simulink model "ClosedLoop_Test"  (R2024a)
settings: Solver=VariableStepAuto  StartTime=0.0  StopTime=10.0  RelTol=1e-3
libraries: RCTblocks x7
settings Model: Creator=Thoma  LastModifiedBy=Thoma

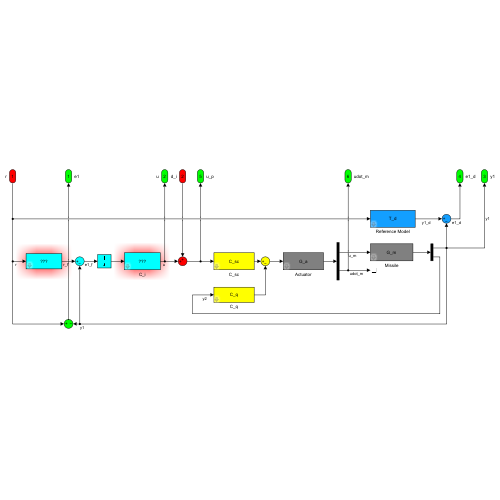
[thumbnail: Simulink's stored preview of the top-level diagram]
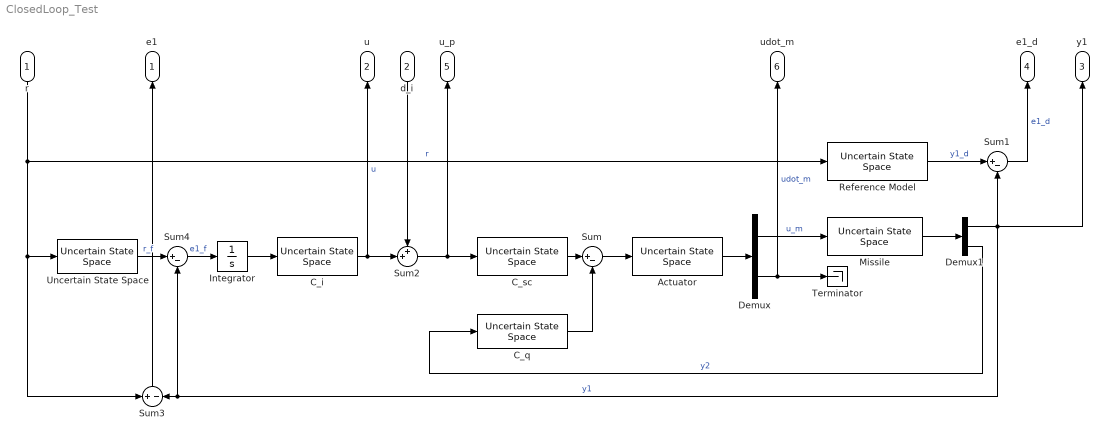
== system ClosedLoop_Test ==
  r : Inport
  d_i : Inport  Port=2
  Actuator : RCTblocks/Uncertain State Space  Tag=USS  USystem=G_a  UValue=[]  X0=[]  uX0=[]
  C_i : RCTblocks/Uncertain State Space  Tag=USS  USystem=C_i  UValue=[]  X0=[]  uX0=[]
  C_q : RCTblocks/Uncertain State Space  Tag=USS  USystem=C_q  UValue=[]  X0=[]  uX0=[]
  C_sc : RCTblocks/Uncertain State Space  Tag=USS  USystem=C_sc  UValue=[]  X0=[]  uX0=[]
  Demux : Demux  Outputs=2
  Demux1 : Demux  Outputs=2
  Integrator : Integrator
  Missile : RCTblocks/Uncertain State Space  Tag=USS  USystem=G_m  UValue=[]  X0=[]  uX0=[]
  Reference Model : RCTblocks/Uncertain State Space  Tag=USS  USystem=T_d  UValue=[]  X0=[]  uX0=[]
  Sum : Sum  Inputs=|+-
  Sum1 : Sum  Inputs=|+-
  Sum2 : Sum  Inputs=++|
  Sum3 : Sum  Inputs=+-
  Sum4 : Sum  Inputs=|+-
  Terminator : Terminator
  Uncertain State Space : RCTblocks/Uncertain State Space  Tag=USS  USystem=F_f  UValue=[]  X0=[]  uX0=[]
  e1 : Outport
  u : Outport  Port=2
  y1 : Outport  Port=3
  e1_d : Outport  Port=4
  u_p : Outport  Port=5
  udot_m : Outport  Port=6
  wires:
  Integrator/1 -> C_i/1
  Demux/2 -> Terminator/1, udot_m/1  "udot_m"
  Demux1/1 -> y1/1, Sum3/2, Sum4/2, Sum1/2  "y1"
  Demux1/2 -> C_q/1  "y2"
  Actuator/1 -> Demux/1
  Missile/1 -> Demux1/1
  C_q/1 -> Sum/2
  C_sc/1 -> Sum/1
  Demux/1 -> Missile/1  "u_m"
  Reference Model/1 -> Sum1/1  "y1_d"
  Sum1/1 -> e1_d/1  "e1_d"
  C_i/1 -> u/1, Sum2/2  "u"
  Sum2/1 -> u_p/1, C_sc/1
  d_i/1 -> Sum2/1
  Sum4/1 -> Integrator/1  "e1_f"
  Uncertain State Space/1 -> Sum4/1  "r_f"
  Sum/1 -> Actuator/1
  Sum3/1 -> e1/1
  r/1 -> Reference Model/1, Sum3/1, Uncertain State Space/1  "r"
